simulink subsystem "GenerateDisturbances"  (R2024a)
settings: Solver=VariableStepAuto  StartTime=0.0  StopTime=10.0  RelTol=1e-3
model mask{max_a=9.81 * Param_ExternalDisturbances_MaxAcceleration(1), T=Param_ExternalDisturbances_AccelerationPeriod(1), t_start=0.5, t_end=1}
  mask prompts: max_a "Max acceleration (m/s^2)"; T "Period (s)"; t_start "Start time (s)"; t_end "Stop time (s)"
undefined symbols (not defined in the file): MCU_Ts, p0
libraries: simulink x1, dspsigops x1
settings Model: Creator=upattacini  LastModifiedBy=upattacini

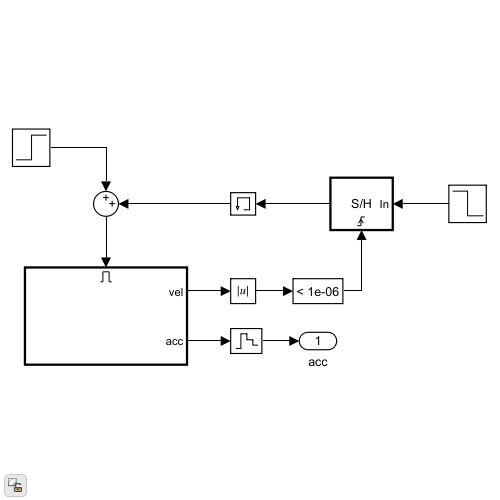
[thumbnail: Simulink's stored preview of the top-level diagram]
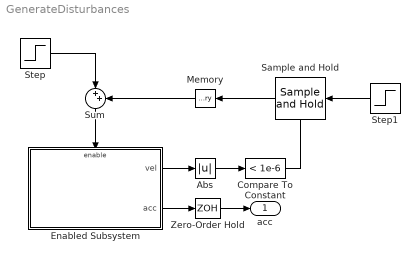
== system GenerateDisturbances ==
  Abs : Abs  RequirementInfo={} %GIDa_75f76463_879e_48e9_8165_53a0db7ed7ec  SaturateOnIntegerOverflow=off
  Compare To Constant : simulink/Logic and Bit Operations/Compare To Constant  relop=<  const=1e-6  OutDataTypeStr=boolean
  Enabled Subsystem : Subsystem  RequirementInfo={} %GIDa_d7277380_fc92_4873_b286_23e089e64faa  TreatAsAtomicUnit=on
  Memory : Memory  RequirementInfo={} %GIDa_0460126a_798a_4bb5_8b23_68e45e869744
  Sample and Hold : dspsigops/Sample and Hold  trig=Rising edge  initCond=0  latchinput=off
  Step : Step  RequirementInfo={} %GIDa_db633ebf_a744_4a81_af60_2985a6487f32  Time=t_start  SampleTime=0
  Step1 : Step  RequirementInfo={} %GIDa_1eae5449_a428_420c_805e_60462c446896  Time=t_end  After=-1  SampleTime=0
  Sum : Sum  RequirementInfo={} %GIDa_a00960e1_2a78_4867_911e_b70e3bbbfbf9  Inputs=|++
  Zero-Order Hold : ZeroOrderHold  RequirementInfo={} %GIDa_5901e23b_4497_4c4a_9d8f_60368a731730  SampleTime=MCU_Ts
  acc : Outport  RequirementInfo={} %GIDa_dee66935_bf33_4a7c_ba62_c3c14f4946c6
  wires:
  Sum/1 -> Enabled Subsystem/Enable
  Enabled Subsystem/2(acc) -> Zero-Order Hold/1
  Zero-Order Hold/1 -> acc/1
  Step/1 -> Sum/1
  Enabled Subsystem/1(vel) -> Abs/1
  Abs/1 -> Compare To Constant/1
  Memory/1 -> Sum/2
  Sample and Hold/1 -> Memory/1
  Compare To Constant/1 -> Sample and Hold/Trigger
  Step1/1 -> Sample and Hold/1

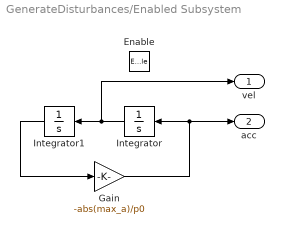
== system GenerateDisturbances/Enabled Subsystem ==
  Enable : EnablePort  RequirementInfo={} %GIDa_32a4d7b0_a0ed_4218_8602_9993c712705a  StatesWhenEnabling=reset
  Gain : Gain  RequirementInfo={} %GIDa_7906ee9f_f9b2_42da_a1b5_7f118fa4c574  Gain=-abs(max_a)/p0
  Integrator : Integrator  RequirementInfo={} %GIDa_a4e3dc54_e490_4950_a5e7_0147b118fe0b
  Integrator1 : Integrator  RequirementInfo={} %GIDa_4fa9565a_634d_45a8_b37a_00e7a8ee875b  InitialCondition=-p0
  vel : Outport  RequirementInfo={} %GIDa_9e7f6d46_db08_4d0a_96c9_c6a196459bcd  OutputWhenDisabled=reset  InitialOutput=0
  acc : Outport  RequirementInfo={} %GIDa_6e1bcf44_7dbe_43ee_8012_64f29cc259e3  Port=2  OutputWhenDisabled=reset  InitialOutput=0
  wires:
  Integrator/1 -> Integrator1/1, vel/1
  Integrator1/1 -> Gain/1
  Gain/1 -> acc/1, Integrator/1
